simulink model "sampleModel7424_pp_1_1"  (R2018a)
settings: Solver=VariableStepAuto  StartTime=0.0  StopTime=10.0  RelTol=1e-3
undefined symbols (not defined in the file): DiscIntNeverNeededParam
libraries: simulink x211
(part 3 of 7)

== system sampleModel7424_pp_1_1/cfblk137 ==
  cfblk1 : Inport
  Action Port : ActionPort  ActionType=then
  cfblk10 : simulink/Discrete/Transfer Fcn Lead or Lag  PoleZ=0.95  ZeroZ=0.75  ICPrevOutput=0.0  ICPrevInput=0.0  DoSatur=off
      settings: SourceProductName=Simulink  SourceProductBaseCode=SL
  cfblk15 : Delay
  cfblk16 : Delay
  cfblk17 : DataTypeConversion  OutDataTypeStr=double
  cfblk18 : DataTypeConversion  OutDataTypeStr=double
  cfblk3 : Delay
  cfblk4 : DiscreteTransferFcn
  cfblk5 : DiscreteFilter
  cfblk6 : simulink/Discrete/Transfer Fcn Lead or Lag  PoleZ=0.95  ZeroZ=0.75  ICPrevOutput=0.0  ICPrevInput=0.0  DoSatur=off
      settings: SourceProductName=Simulink  SourceProductBaseCode=SL
  cfblk7 : Delay  DelayLengthSource=Input port
      settings: InputPortMap=u0,p1
  cfblk8 : simulink/Discrete/Tapped Delay  vinit=0.0  samptime=-1  NumDelays=1  DelayOrder=Oldest  includeCurrent=off
  cfblk9 : Delay  DelayLengthSource=Input port
      settings: InputPortMap=u0,p1
  cyemi_{473,475..476,479..482,485} (8 alike) : DataTypeConversion  OutDataTypeStr=double
  cyemi_{474,477..478,483..484,486} (6 alike) : DataTypeConversion  OutDataTypeStr=uint32
  cfblk2 : Outport
  cfblk11 : Outport  Port=2
  cfblk12 : Outport  Port=3
  cfblk13 : Outport  Port=4
  cfblk14 : Outport  Port=5
  wires:
  cfblk9/1 -> cfblk11/1, cyemi_482/1
  cfblk7/1 -> cfblk12/1
  cfblk6/1 -> cyemi_473/1, cyemi_485/1
  cfblk1/1 -> cfblk13/1
  cfblk3/1 -> cfblk14/1, cyemi_484/1
  cfblk8/1 -> cyemi_474/1, cyemi_477/1, cyemi_483/1, cyemi_486/1
  cfblk17/1 -> cfblk2/1
  cyemi_473/1 -> cfblk10/1
  cyemi_474/1 -> cfblk15/1
  cyemi_475/1 -> cfblk16/1
  cfblk10/1 -> cyemi_475/1
  cyemi_476/1 -> cfblk17/1
  cfblk4/1 -> cyemi_476/1
  cyemi_477/1 -> cfblk18/1
  cyemi_478/1 -> cfblk3/1
  cfblk15/1 -> cyemi_478/1
  cyemi_479/1 -> cfblk4/1
  cfblk18/1 -> cyemi_479/1
  cyemi_480/1 -> cfblk5/1
  cfblk16/1 -> cyemi_480/1
  cyemi_481/1 -> cfblk6/1
  cfblk5/1 -> cyemi_481/1
  cyemi_482/1 -> cfblk7/1
  cyemi_483/1 -> cfblk7/2
  cyemi_484/1 -> cfblk8/1
  cyemi_485/1 -> cfblk9/1
  cyemi_486/1 -> cfblk9/2

== system sampleModel7424_pp_1_1/cfblk138 ==
  cfblk1 : Inport
  cfblk6 : Inport  Port=2
  Action Port : ActionPort  ActionType=else
  cfblk3 : DiscreteTransferFcn
  cfblk4 : simulink/Continuous/PID Controller (2DOF)  Controller=PID  TimeDomain=Discrete-time  SampleTime=-1  IntegratorMethod=Forward Euler  FilterMethod=Forward Euler  Form=Parallel  UseFilter=on  ControllerParametersSource=internal  P=1  I=1  D=0  N=100  b=1  c=1  InitialConditionSource=internal  InitialConditionForIntegrator=0  InitialConditionForFilter=0  ExternalReset=none  LimitOutput=off  UpperSaturationLimit=inf  LowerSaturationLimit=-inf  LinearizeAsGain=off  AntiWindupMode=none  Kb=1  TrackingMode=off  Kt=1  PParamMin=[]  PParamMax=[]  IParamMin=[]  IParamMax=[]  DParamMin=[]  DParamMax=[]  NParamMin=[]  NParamMax=[]  bParamMin=[]  bParamMax=[]  cParamMin=[]  cParamMax=[]  KbParamMin=[]  KbParamMax=[]  KtParamMin=[]  KtParamMax=[]  POutMin=[]  POutMax=[]  IOutMin=[]  IOutMax=[]  DOutMin=[]  DOutMax=[]  NOutMin=[]  NOutMax=[]  bOutMin=[]  bOutMax=[]  cOutMin=[]  cOutMax=[]  KbOutMin=[]  KbOutMax=[]  KtOutMin=[]  KtOutMax=[]  IntegratorOutMin=[]  IntegratorOutMax=[]  FilterOutMin=[]  FilterOutMax=[]  SumOutMin=[]  SumOutMax=[]  Sum1OutMin=[]  Sum1OutMax=[]  Sum2OutMin=[]  Sum2OutMax=[]  Sum3OutMin=[]  Sum3OutMax=[]  SumI1OutMin=[]  SumI1OutMax=[]  SumI2OutMin=[]  SumI2OutMax=[]  SumI3OutMin=[]  SumI3OutMax=[]  SumDOutMin=[]  SumDOutMax=[]  SaturationOutMin=[]  SaturationOutMax=[]  IntegratorContinuousStateAttributes=''  IntegratorStateMustResolveToSignalObject=off  IntegratorRTWStateStorageClass=Auto  FilterContinuousStateAttributes=''  FilterStateMustResolveToSignalObject=off  FilterRTWStateStorageClass=Auto  DifferentiatorICPrevScaledInput=0  DifferentiatorOutMin=[]  DifferentiatorOutMax=[]  FilterDiffOutCoefMin=[]  FilterDiffOutCoefMax=[]  SumDenOutMin=[]  SumDenOutMax=[]  SumNumOutMin=[]  SumNumOutMax=[]  ReciprocalOutMin=[]  ReciprocalOutMax=[]  DivideOutMin=[]  DivideOutMax=[]  TunerSelectOption=Transfer Function Based (PID Tuner App)
  cfblk5 : DiscreteFilter
  cyemi_{489..492} (4 alike) : DataTypeConversion  OutDataTypeStr=double
  emi_{144,174,244,296} (4 alike) : UnaryMinus
  emi_145 : MATLAB Function  TreatAsAtomicUnit=on
  emi_175 : MATLAB Function  TreatAsAtomicUnit=on
  emi_245 : MATLAB Function  TreatAsAtomicUnit=on
  emi_297 : MATLAB Function  TreatAsAtomicUnit=on
  cfblk2 : Outport
  cfblk7 : Outport  Port=2
  wires:
  cfblk1/1 -> cfblk2/1
  cfblk5/1 -> cfblk7/1
  cyemi_489/1 -> cfblk3/1, emi_144/1, emi_145/1(o), emi_174/1, emi_175/1(o)
  cfblk4/1 -> cyemi_489/1
  cyemi_490/1 -> cfblk4/1, emi_296/1, emi_297/1(o)
  cfblk6/1 -> cyemi_490/1, cyemi_491/1
  cyemi_491/1 -> cfblk4/2
  cyemi_492/1 -> cfblk5/1, emi_244/1, emi_245/1(o)
  cfblk3/1 -> cyemi_492/1
  emi_144/1 -> emi_145/2(e)
  emi_174/1 -> emi_175/2(e)
  emi_244/1 -> emi_245/2(e)
  emi_296/1 -> emi_297/2(e)

== system sampleModel7424_pp_1_1/cfblk139 ==
  cfblk1 : Inport
  cfblk8 : Inport  Port=2
  Action Port : ActionPort  ActionType=then
  cfblk3 : DiscreteZeroPole  Poles=[0 0.5]  Gain=1  SampleTime=-1
  cfblk4 : DiscreteTransferFcn
  cfblk5 : DiscreteIntegrator  SampleTime=-1  OutDataTypeStr=double  ICPrevOutput=DiscIntNeverNeededParam  ICPrevScaledInput=DiscIntNeverNeededParam
  cfblk6 : simulink/Discrete/Tapped Delay  vinit=0.0  samptime=-1  NumDelays=1  DelayOrder=Oldest  includeCurrent=off
  cfblk7 : simulink/Discrete/Difference  ICPrevInput=0.0  OutMin=[]  OutMax=[]  OutDataTypeStr=double  OutputDataTypeScalingMode=double  OutDataType=fixdt(1, 16)  OutScaling=2^-10  DoSatur=off
  cyemi_{495..499} (5 alike) : DataTypeConversion  OutDataTypeStr=double
  cfblk2 : Outport
  cfblk9 : Outport  Port=2
  cfblk10 : Outport  Port=3
  wires:
  cfblk4/1 -> cyemi_495/1, cyemi_499/1
  cfblk3/1 -> cfblk9/1
  cfblk8/1 -> cfblk2/1
  cfblk7/1 -> cfblk10/1
  cyemi_495/1 -> cfblk3/1
  cyemi_496/1 -> cfblk4/1
  cfblk5/1 -> cyemi_496/1
  cyemi_497/1 -> cfblk5/1
  cfblk6/1 -> cyemi_497/1
  cyemi_498/1 -> cfblk6/1
  cfblk1/1 -> cyemi_498/1
  cyemi_499/1 -> cfblk7/1

== system sampleModel7424_pp_1_1/cfblk140 ==
  cfblk1 : Inport
  Action Port : ActionPort  ActionType=else
  cfblk3 : Delay
  cfblk4 : simulink/Discrete/Transfer Fcn First Order  PoleZ=0.95  ICPrevOutput=0.0  DoSatur=off
      settings: SourceProductName=Simulink
  cfblk5 : Delay  ShowEnablePort=on
      settings: InputPortMap=u0,e6
  cfblk6 : Delay  ShowEnablePort=on
      settings: InputPortMap=u0,e6
  cyemi_{502..507} (6 alike) : DataTypeConversion  OutDataTypeStr=double
  emi_118 : UnaryMinus
  emi_119 : MATLAB Function  TreatAsAtomicUnit=on
  emi_270 : UnaryMinus
  emi_271 : MATLAB Function  TreatAsAtomicUnit=on
  emi_304 : UnaryMinus
  emi_305 : MATLAB Function  TreatAsAtomicUnit=on
  cfblk2 : Outport
  cfblk7 : Outport  Port=2
  cfblk8 : Outport  Port=3
  wires:
  cfblk4/1 -> cyemi_505/1, cyemi_506/1
  cfblk3/1 -> cyemi_504/1, cyemi_507/1
  cfblk6/1 -> cfblk2/1
  cfblk1/1 -> cyemi_502/1, cyemi_503/1
  cfblk5/1 -> cfblk8/1, cfblk7/1
  cyemi_502/1 -> cfblk3/1, emi_118/1, emi_119/1(o), emi_270/1, emi_271/1(o)
  cyemi_503/1 -> cfblk4/1, emi_304/1, emi_305/1(o)
  cyemi_504/1 -> cfblk5/1
  cyemi_505/1 -> cfblk5/2
  cyemi_506/1 -> cfblk6/1
  cyemi_507/1 -> cfblk6/2
  emi_118/1 -> emi_119/2(e)
  emi_270/1 -> emi_271/2(e)
  emi_304/1 -> emi_305/2(e)

== system sampleModel7424_pp_1_1/cfblk141 ==
  cfblk1 : Inport
  cfblk13 : Inport  Port=2
  cfblk14 : Inport  Port=3
  Action Port : ActionPort  ActionType=then
  cfblk10 : DiscreteFilter
  cfblk11 : simulink/Discrete/Transfer Fcn Lead or Lag  PoleZ=0.95  ZeroZ=0.75  ICPrevOutput=0.0  ICPrevInput=0.0  DoSatur=off
      settings: SourceProductName=Simulink  SourceProductBaseCode=SL
  cfblk12 : simulink/Discrete/Transfer Fcn First Order  PoleZ=0.95  ICPrevOutput=0.0  DoSatur=off
      settings: SourceProductName=Simulink
  cfblk3 : DiscreteIntegrator  SampleTime=-1  OutDataTypeStr=double  ICPrevOutput=DiscIntNeverNeededParam  ICPrevScaledInput=DiscIntNeverNeededParam
  cfblk4 : simulink/Discrete/Transfer Fcn Lead or Lag  PoleZ=0.95  ZeroZ=0.75  ICPrevOutput=0.0  ICPrevInput=0.0  DoSatur=off
      settings: SourceProductName=Simulink  SourceProductBaseCode=SL
  cfblk5 : DiscreteIntegrator  SampleTime=-1  OutDataTypeStr=double  ICPrevOutput=DiscIntNeverNeededParam  ICPrevScaledInput=DiscIntNeverNeededParam
  cfblk6 : simulink/Discrete/Transfer Fcn First Order  PoleZ=0.95  ICPrevOutput=0.0  DoSatur=off
      settings: SourceProductName=Simulink
  cfblk7 : simulink/Continuous/PID Controller  Controller=PID  TimeDomain=Discrete-time  SampleTime=-1  IntegratorMethod=Forward Euler  FilterMethod=Forward Euler  Form=Parallel  UseFilter=on  ControllerParametersSource=internal  P=1  I=1  D=0  N=100  InitialConditionSource=internal  InitialConditionForIntegrator=0  InitialConditionForFilter=0  ExternalReset=none  LimitOutput=off  UpperSaturationLimit=inf  LowerSaturationLimit=-inf  LinearizeAsGain=off  AntiWindupMode=none  Kb=1  TrackingMode=off  Kt=1  PParamMin=[]  PParamMax=[]  IParamMin=[]  IParamMax=[]  DParamMin=[]  DParamMax=[]  NParamMin=[]  NParamMax=[]  KbParamMin=[]  KbParamMax=[]  KtParamMin=[]  KtParamMax=[]  POutMin=[]  POutMax=[]  IOutMin=[]  IOutMax=[]  DOutMin=[]  DOutMax=[]  NOutMin=[]  NOutMax=[]  KbOutMin=[]  KbOutMax=[]  KtOutMin=[]  KtOutMax=[]  IntegratorOutMin=[]  IntegratorOutMax=[]  FilterOutMin=[]  FilterOutMax=[]  SumOutMin=[]  SumOutMax=[]  SumI1OutMin=[]  SumI1OutMax=[]  SumI2OutMin=[]  SumI2OutMax=[]  SumI3OutMin=[]  SumI3OutMax=[]  SumDOutMin=[]  SumDOutMax=[]  SaturationOutMin=[]  SaturationOutMax=[]  IntegratorContinuousStateAttributes=''  IntegratorStateMustResolveToSignalObject=off  IntegratorRTWStateStorageClass=Auto  FilterContinuousStateAttributes=''  FilterStateMustResolveToSignalObject=off  FilterRTWStateStorageClass=Auto  DifferentiatorICPrevScaledInput=0  DifferentiatorOutMin=[]  DifferentiatorOutMax=[]  FilterDiffOutCoefMin=[]  FilterDiffOutCoefMax=[]  SumDenOutMin=[]  SumDenOutMax=[]  SumNumOutMin=[]  SumNumOutMax=[]  ReciprocalOutMin=[]  ReciprocalOutMax=[]  DivideOutMin=[]  DivideOutMax=[]  TunerSelectOption=Transfer Function Based (PID Tuner App)
  cfblk8 : simulink/Discrete/Transfer Fcn Real Zero  ZeroZ=0.75  ICPrevInput=0.0  DoSatur=off
      settings: SourceProductName=Simulink  SourceProductBaseCode=SL
  cfblk9 : DiscreteZeroPole  Poles=[0 0.5]  Gain=1  SampleTime=-1
  cyemi_{511..520} (10 alike) : DataTypeConversion  OutDataTypeStr=double
  emi_{142,216,242,262} (4 alike) : UnaryMinus
  emi_143 : MATLAB Function  TreatAsAtomicUnit=on
  emi_217 : MATLAB Function  TreatAsAtomicUnit=on
  emi_243 : MATLAB Function  TreatAsAtomicUnit=on
  emi_263 : MATLAB Function  TreatAsAtomicUnit=on
  cfblk2 : Outport
  wires:
  cfblk12/1 -> cfblk2/1
  cyemi_511/1 -> cfblk10/1, emi_142/1, emi_143/1(o)
  cfblk4/1 -> cyemi_511/1
  cyemi_512/1 -> cfblk11/1
  cfblk7/1 -> cyemi_512/1
  cyemi_513/1 -> cfblk12/1
  cfblk13/1 -> cyemi_513/1
  cyemi_514/1 -> cfblk3/1
  cfblk9/1 -> cyemi_514/1
  cyemi_515/1 -> cfblk4/1
  cfblk6/1 -> cyemi_515/1
  cyemi_516/1 -> cfblk5/1, emi_242/1, emi_243/1(o)
  cfblk11/1 -> cyemi_516/1
  cyemi_517/1 -> cfblk6/1, emi_216/1, emi_217/1(o)
  cfblk14/1 -> cyemi_517/1
  cyemi_518/1 -> cfblk7/1
  cfblk10/1 -> cyemi_518/1
  cyemi_519/1 -> cfblk8/1, emi_262/1, emi_263/1(o)
  cfblk3/1 -> cyemi_519/1
  cyemi_520/1 -> cfblk9/1
  cfblk1/1 -> cyemi_520/1
  emi_142/1 -> emi_143/2(e)
  emi_216/1 -> emi_217/2(e)
  emi_242/1 -> emi_243/2(e)
  emi_262/1 -> emi_263/2(e)

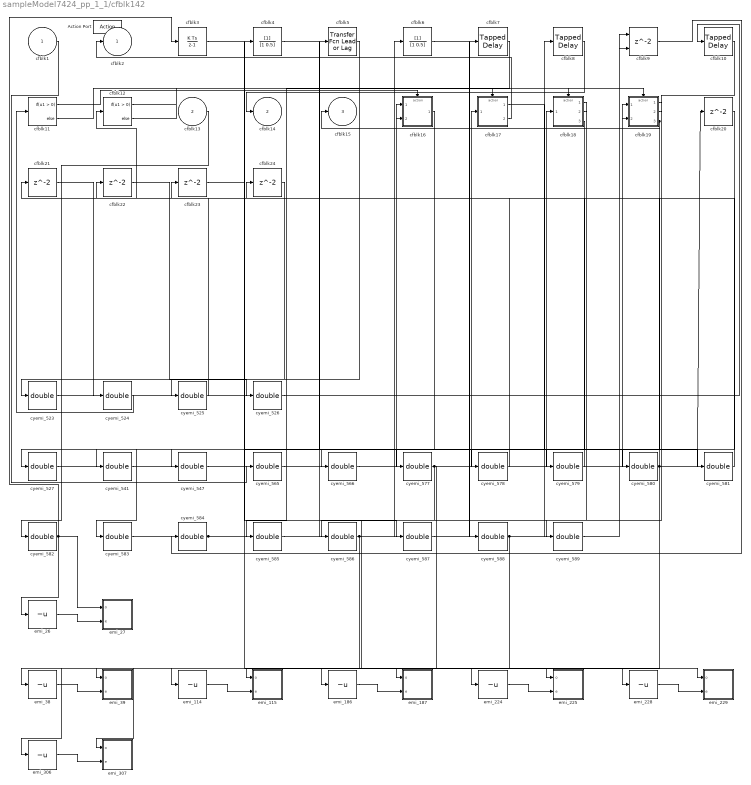
== system sampleModel7424_pp_1_1/cfblk142 ==
  cfblk1 : Inport
  cfblk13 : Inport  Port=2
  Action Port : ActionPort  ActionType=else
  cfblk10 : simulink/Discrete/Tapped Delay  vinit=0.0  samptime=-1  NumDelays=1  DelayOrder=Oldest  includeCurrent=off
  cfblk11 : If  SampleTime=1
  cfblk12 : If  SampleTime=1
  cfblk16 : Subsystem  TreatAsAtomicUnit=on
  cfblk17 : Subsystem  TreatAsAtomicUnit=on
  cfblk18 : Subsystem  TreatAsAtomicUnit=on
  cfblk19 : Subsystem  TreatAsAtomicUnit=on
  cfblk{20..24} (5 alike) : Delay
  cfblk3 : DiscreteIntegrator  SampleTime=-1  OutDataTypeStr=double  ICPrevOutput=DiscIntNeverNeededParam  ICPrevScaledInput=DiscIntNeverNeededParam
  cfblk4 : DiscreteFilter
  cfblk5 : simulink/Discrete/Transfer Fcn Lead or Lag  PoleZ=0.95  ZeroZ=0.75  ICPrevOutput=0.0  ICPrevInput=0.0  DoSatur=off
      settings: SourceProductName=Simulink  SourceProductBaseCode=SL
  cfblk6 : DiscreteFilter
  cfblk7 : simulink/Discrete/Tapped Delay  vinit=0.0  samptime=-1  NumDelays=1  DelayOrder=Oldest  includeCurrent=off
  cfblk8 : simulink/Discrete/Tapped Delay  vinit=0.0  samptime=-1  NumDelays=1  DelayOrder=Oldest  includeCurrent=off
  cfblk9 : Delay  ShowEnablePort=on
      settings: InputPortMap=u0,e6
  cyemi_{523..527,541,547,565..566,577..589} (22 alike) : DataTypeConversion  OutDataTypeStr=double
  emi_{26,38,114,186,224,228,306} (7 alike) : UnaryMinus
  emi_115 : MATLAB Function  TreatAsAtomicUnit=on
  emi_187 : MATLAB Function  TreatAsAtomicUnit=on
  emi_225 : MATLAB Function  TreatAsAtomicUnit=on
  emi_229 : MATLAB Function  TreatAsAtomicUnit=on
  emi_27 : MATLAB Function  TreatAsAtomicUnit=on
  emi_307 : MATLAB Function  TreatAsAtomicUnit=on
  emi_39 : MATLAB Function  TreatAsAtomicUnit=on
  cfblk2 : Outport
  cfblk14 : Outport  Port=2
  cfblk15 : Outport  Port=3
  wires:
  cfblk8/1 -> cfblk14/1
  cfblk19/3(cfblk13) -> cfblk15/1, cyemi_582/1
  cfblk17/2(cfblk7) -> cfblk2/1
  cfblk11/1 -> cfblk16/Action
  cfblk11/2 -> cfblk17/Action
  cfblk12/1 -> cfblk18/Action
  cfblk12/2 -> cfblk19/Action
  cyemi_523/1 -> cfblk10/1
  cfblk5/1 -> cyemi_523/1
  cyemi_524/1 -> cfblk11/1
  cfblk21/1 -> cyemi_524/1
  cyemi_525/1 -> cfblk12/1
  cfblk24/1 -> cyemi_525/1
  cyemi_526/1 -> cfblk16/1(cfblk1)
  cfblk22/1 -> cyemi_526/1
  cyemi_527/1 -> cfblk16/2(cfblk11)
  cfblk13/1 -> cyemi_527/1
  cyemi_541/1 -> cfblk17/1(cfblk1)
  cfblk19/1(cfblk2) -> cyemi_541/1
  cyemi_547/1 -> cfblk18/1(cfblk1)
  cfblk20/1 -> cyemi_547/1
  cyemi_565/1 -> cfblk19/1(cfblk1)
  cfblk1/1 -> cyemi_565/1
  cyemi_566/1 -> cfblk19/2(cfblk11)
  cfblk23/1 -> cyemi_566/1
  cyemi_577/1 -> cfblk20/1, emi_186/1, emi_187/1(o)
  cfblk16/1(cfblk2) -> cyemi_577/1
  cyemi_578/1 -> cfblk21/1
  cfblk10/1 -> cyemi_578/1
  cyemi_579/1 -> cfblk22/1
  cfblk18/2(cfblk14) -> cyemi_579/1
  cyemi_580/1 -> cfblk23/1, emi_224/1, emi_225/1(o), emi_306/1, emi_307/1(o)
  cfblk4/1 -> cyemi_580/1
  cyemi_581/1 -> cfblk24/1
  cfblk17/1(cfblk2) -> cyemi_581/1
  cyemi_582/1 -> cfblk3/1, emi_26/1, emi_27/1(o)
  cyemi_583/1 -> cfblk4/1
  cfblk18/3(cfblk15) -> cyemi_583/1
  cyemi_584/1 -> cfblk5/1, emi_228/1, emi_229/1(o)
  cfblk9/1 -> cyemi_584/1
  cyemi_585/1 -> cfblk6/1
  cfblk7/1 -> cyemi_585/1
  cyemi_586/1 -> cfblk7/1, emi_114/1, emi_115/1(o)
  cfblk19/2(cfblk12) -> cyemi_586/1
  cyemi_587/1 -> cfblk8/1
  cfblk3/1 -> cyemi_587/1
  cyemi_588/1 -> cfblk9/1, emi_38/1, emi_39/1(o)
  cfblk6/1 -> cyemi_588/1
  cyemi_589/1 -> cfblk9/2
  cfblk18/1(cfblk2) -> cyemi_589/1
  emi_26/1 -> emi_27/2(e)
  emi_38/1 -> emi_39/2(e)
  emi_114/1 -> emi_115/2(e)
  emi_186/1 -> emi_187/2(e)
  emi_224/1 -> emi_225/2(e)
  emi_228/1 -> emi_229/2(e)
  emi_306/1 -> emi_307/2(e)

== system sampleModel7424_pp_1_1/cfblk143 ==
  cfblk1 : Inport
  Action Port : ActionPort  ActionType=then
  cfblk3 : UnitDelay  SampleTime=-1
  cfblk4 : DiscreteZeroPole  Poles=[0 0.5]  Gain=1  SampleTime=-1
  cfblk5 : DiscreteZeroPole  Poles=[0 0.5]  Gain=1  SampleTime=-1
  cfblk6 : simulink/Discrete/Transfer Fcn First Order  PoleZ=0.95  ICPrevOutput=0.0  DoSatur=off
      settings: SourceProductName=Simulink
  cfblk7 : DiscreteZeroPole  Poles=[0 0.5]  Gain=1  SampleTime=-1
  cfblk8 : Delay
  cfblk9 : DataTypeConversion  OutDataTypeStr=double
  cyemi_{591..596} (6 alike) : DataTypeConversion  OutDataTypeStr=double
  cyemi_597 : DataTypeConversion  OutDataTypeStr=uint16
  cfblk2 : Outport
  wires:
  cfblk7/1 -> cfblk2/1
  cyemi_591/1 -> cfblk3/1
  cfblk8/1 -> cyemi_591/1
  cyemi_592/1 -> cfblk4/1
  cfblk6/1 -> cyemi_592/1
  cyemi_593/1 -> cfblk5/1
  cfblk4/1 -> cyemi_593/1
  cyemi_594/1 -> cfblk6/1
  cfblk3/1 -> cyemi_594/1
  cyemi_595/1 -> cfblk7/1
  cfblk9/1 -> cyemi_595/1
  cyemi_596/1 -> cfblk8/1
  cfblk5/1 -> cyemi_596/1
  cyemi_597/1 -> cfblk9/1
  cfblk1/1 -> cyemi_597/1

== system sampleModel7424_pp_1_1/cfblk144 ==
  cfblk1 : Inport
  cfblk12 : Inport  Port=2
  cfblk13 : Inport  Port=3
  Action Port : ActionPort  ActionType=else
  cfblk10 : simulink/Continuous/PID Controller  Controller=PID  TimeDomain=Discrete-time  SampleTime=-1  IntegratorMethod=Forward Euler  FilterMethod=Forward Euler  Form=Parallel  UseFilter=on  ControllerParametersSource=internal  P=1  I=1  D=0  N=100  InitialConditionSource=internal  InitialConditionForIntegrator=0  InitialConditionForFilter=0  ExternalReset=none  LimitOutput=off  UpperSaturationLimit=inf  LowerSaturationLimit=-inf  LinearizeAsGain=off  AntiWindupMode=none  Kb=1  TrackingMode=off  Kt=1  PParamMin=[]  PParamMax=[]  IParamMin=[]  IParamMax=[]  DParamMin=[]  DParamMax=[]  NParamMin=[]  NParamMax=[]  KbParamMin=[]  KbParamMax=[]  KtParamMin=[]  KtParamMax=[]  POutMin=[]  POutMax=[]  IOutMin=[]  IOutMax=[]  DOutMin=[]  DOutMax=[]  NOutMin=[]  NOutMax=[]  KbOutMin=[]  KbOutMax=[]  KtOutMin=[]  KtOutMax=[]  IntegratorOutMin=[]  IntegratorOutMax=[]  FilterOutMin=[]  FilterOutMax=[]  SumOutMin=[]  SumOutMax=[]  SumI1OutMin=[]  SumI1OutMax=[]  SumI2OutMin=[]  SumI2OutMax=[]  SumI3OutMin=[]  SumI3OutMax=[]  SumDOutMin=[]  SumDOutMax=[]  SaturationOutMin=[]  SaturationOutMax=[]  IntegratorContinuousStateAttributes=''  IntegratorStateMustResolveToSignalObject=off  IntegratorRTWStateStorageClass=Auto  FilterContinuousStateAttributes=''  FilterStateMustResolveToSignalObject=off  FilterRTWStateStorageClass=Auto  DifferentiatorICPrevScaledInput=0  DifferentiatorOutMin=[]  DifferentiatorOutMax=[]  FilterDiffOutCoefMin=[]  FilterDiffOutCoefMax=[]  SumDenOutMin=[]  SumDenOutMax=[]  SumNumOutMin=[]  SumNumOutMax=[]  ReciprocalOutMin=[]  ReciprocalOutMax=[]  DivideOutMin=[]  DivideOutMax=[]  TunerSelectOption=Transfer Function Based (PID Tuner App)
  cfblk11 : Delay  DelayLengthSource=Input port
      settings: InputPortMap=u0,p1
  cfblk14 : Delay
  cfblk3 : simulink/Discrete/Tapped Delay  vinit=0.0  samptime=-1  NumDelays=1  DelayOrder=Oldest  includeCurrent=off
  cfblk4 : simulink/Continuous/PID Controller  Controller=PID  TimeDomain=Discrete-time  SampleTime=-1  IntegratorMethod=Forward Euler  FilterMethod=Forward Euler  Form=Parallel  UseFilter=on  ControllerParametersSource=internal  P=1  I=1  D=0  N=100  InitialConditionSource=internal  InitialConditionForIntegrator=0  InitialConditionForFilter=0  ExternalReset=none  LimitOutput=off  UpperSaturationLimit=inf  LowerSaturationLimit=-inf  LinearizeAsGain=off  AntiWindupMode=none  Kb=1  TrackingMode=off  Kt=1  PParamMin=[]  PParamMax=[]  IParamMin=[]  IParamMax=[]  DParamMin=[]  DParamMax=[]  NParamMin=[]  NParamMax=[]  KbParamMin=[]  KbParamMax=[]  KtParamMin=[]  KtParamMax=[]  POutMin=[]  POutMax=[]  IOutMin=[]  IOutMax=[]  DOutMin=[]  DOutMax=[]  NOutMin=[]  NOutMax=[]  KbOutMin=[]  KbOutMax=[]  KtOutMin=[]  KtOutMax=[]  IntegratorOutMin=[]  IntegratorOutMax=[]  FilterOutMin=[]  FilterOutMax=[]  SumOutMin=[]  SumOutMax=[]  SumI1OutMin=[]  SumI1OutMax=[]  SumI2OutMin=[]  SumI2OutMax=[]  SumI3OutMin=[]  SumI3OutMax=[]  SumDOutMin=[]  SumDOutMax=[]  SaturationOutMin=[]  SaturationOutMax=[]  IntegratorContinuousStateAttributes=''  IntegratorStateMustResolveToSignalObject=off  IntegratorRTWStateStorageClass=Auto  FilterContinuousStateAttributes=''  FilterStateMustResolveToSignalObject=off  FilterRTWStateStorageClass=Auto  DifferentiatorICPrevScaledInput=0  DifferentiatorOutMin=[]  DifferentiatorOutMax=[]  FilterDiffOutCoefMin=[]  FilterDiffOutCoefMax=[]  SumDenOutMin=[]  SumDenOutMax=[]  SumNumOutMin=[]  SumNumOutMax=[]  ReciprocalOutMin=[]  ReciprocalOutMax=[]  DivideOutMin=[]  DivideOutMax=[]  TunerSelectOption=Transfer Function Based (PID Tuner App)
  cfblk5 : simulink/Discrete/Transfer Fcn Real Zero  ZeroZ=0.75  ICPrevInput=0.0  DoSatur=off
      settings: SourceProductName=Simulink  SourceProductBaseCode=SL
  cfblk6 : DiscreteFir
  cfblk7 : DiscreteFir
  cfblk8 : DiscreteTransferFcn
  cfblk9 : simulink/Discrete/Transfer Fcn Lead or Lag  PoleZ=0.95  ZeroZ=0.75  ICPrevOutput=0.0  ICPrevInput=0.0  DoSatur=off
      settings: SourceProductName=Simulink  SourceProductBaseCode=SL
  cyemi_{601..611} (11 alike) : DataTypeConversion  OutDataTypeStr=double
  emi_196 : UnaryMinus
  emi_197 : MATLAB Function  TreatAsAtomicUnit=on
  cfblk2 : Outport
  wires:
  cfblk12/1 -> cfblk2/1
  cyemi_601/1 -> cfblk10/1
  cfblk5/1 -> cyemi_601/1
  cyemi_602/1 -> cfblk11/1
  cfblk1/1 -> cyemi_602/1
  cyemi_603/1 -> cfblk11/2
  cfblk3/1 -> cyemi_603/1
  cyemi_604/1 -> cfblk14/1
  cfblk7/1 -> cyemi_604/1
  cyemi_605/1 -> cfblk3/1
  cfblk9/1 -> cyemi_605/1
  cyemi_606/1 -> cfblk4/1, emi_196/1, emi_197/1(o)
  cfblk13/1 -> cyemi_606/1
  cyemi_607/1 -> cfblk5/1
  cfblk4/1 -> cyemi_607/1
  cyemi_608/1 -> cfblk6/1
  cfblk14/1 -> cyemi_608/1
  cyemi_609/1 -> cfblk7/1
  cfblk8/1 -> cyemi_609/1
  cyemi_610/1 -> cfblk8/1
  cfblk6/1 -> cyemi_610/1
  cyemi_611/1 -> cfblk9/1
  cfblk10/1 -> cyemi_611/1
  emi_196/1 -> emi_197/2(e)

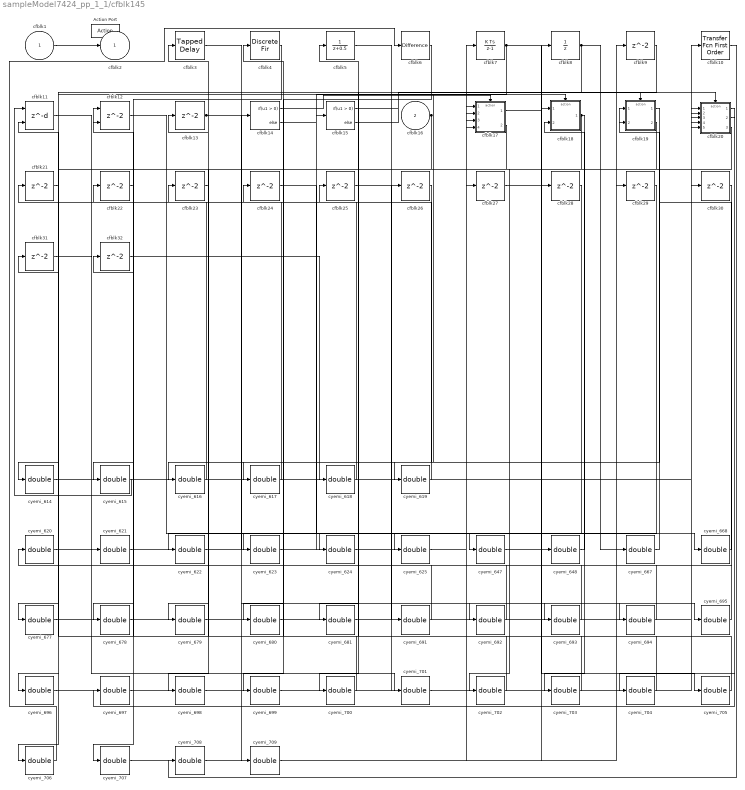
== system sampleModel7424_pp_1_1/cfblk145 ==
  cfblk1 : Inport
  cfblk16 : Inport  Port=2
  Action Port : ActionPort  ActionType=then
  cfblk10 : simulink/Discrete/Transfer Fcn First Order  PoleZ=0.95  ICPrevOutput=0.0  DoSatur=off
      settings: SourceProductName=Simulink
  cfblk11 : Delay  DelayLengthSource=Input port
      settings: InputPortMap=u0,p1
  cfblk12 : Delay  ShowEnablePort=on
      settings: InputPortMap=u0,e6
  cfblk{9,13,21..32} (14 alike) : Delay
  cfblk14 : If  SampleTime=1
  cfblk15 : If  SampleTime=1
  cfblk17 : Subsystem  TreatAsAtomicUnit=on
  cfblk18 : Subsystem  TreatAsAtomicUnit=on
  cfblk19 : Subsystem  TreatAsAtomicUnit=on
  cfblk20 : Subsystem  TreatAsAtomicUnit=on
  cfblk3 : simulink/Discrete/Tapped Delay  vinit=0.0  samptime=-1  NumDelays=1  DelayOrder=Oldest  includeCurrent=off
  cfblk4 : DiscreteFir
  cfblk5 : DiscreteTransferFcn
  cfblk6 : simulink/Discrete/Difference  ICPrevInput=0.0  OutMin=[]  OutMax=[]  OutDataTypeStr=double  OutputDataTypeScalingMode=double  OutDataType=fixdt(1, 16)  OutScaling=2^-10  DoSatur=off
  cfblk7 : DiscreteIntegrator  SampleTime=-1  OutDataTypeStr=double  ICPrevOutput=DiscIntNeverNeededParam  ICPrevScaledInput=DiscIntNeverNeededParam
  cfblk8 : UnitDelay  SampleTime=-1
  cyemi_{614..625,647..648,667..668,677..681,691..709} (40 alike) : DataTypeConversion  OutDataTypeStr=double
  cfblk2 : Outport
  wires:
  cfblk1/1 -> cfblk2/1
  cfblk8/1 -> cyemi_667/1, cyemi_681/1
  cfblk16/1 -> cyemi_615/1, cyemi_680/1
  cfblk13/1 -> cyemi_692/1, cyemi_693/1, cyemi_694/1
  cfblk7/1 -> cyemi_619/1, cyemi_695/1, cyemi_696/1
  cfblk18/1(cfblk2) -> cyemi_614/1, cyemi_624/1, cyemi_703/1
  cfblk14/1 -> cfblk17/Action
  cfblk14/2 -> cfblk18/Action
  cfblk15/1 -> cfblk19/Action
  cfblk15/2 -> cfblk20/Action
  cyemi_614/1 -> cfblk10/1
  cyemi_615/1 -> cfblk11/1
  cyemi_616/1 -> cfblk11/2
  cfblk19/1(cfblk2) -> cyemi_616/1
  cyemi_617/1 -> cfblk12/1
  cfblk6/1 -> cyemi_617/1
  cyemi_618/1 -> cfblk12/2
  cfblk32/1 -> cyemi_618/1
  cyemi_619/1 -> cfblk13/1
  cyemi_620/1 -> cfblk14/1
  cfblk30/1 -> cyemi_620/1
  cyemi_621/1 -> cfblk15/1
  cfblk31/1 -> cyemi_621/1
  cyemi_622/1 -> cfblk17/1(cfblk1)
  cfblk28/1 -> cyemi_622/1
  cyemi_623/1 -> cfblk17/2(cfblk14)
  cfblk26/1 -> cyemi_623/1
  cyemi_624/1 -> cfblk17/3(cfblk15)
  cyemi_625/1 -> cfblk17/4(cfblk16)
  cfblk24/1 -> cyemi_625/1
  cyemi_647/1 -> cfblk18/1(cfblk1)
  cfblk12/1 -> cyemi_647/1
  cyemi_648/1 -> cfblk18/2(cfblk15)
  cfblk27/1 -> cyemi_648/1
  cyemi_667/1 -> cfblk19/1(cfblk1)
  cyemi_668/1 -> cfblk19/2(cfblk11)
  cfblk25/1 -> cyemi_668/1
  cyemi_677/1 -> cfblk20/1(cfblk1)
  cfblk21/1 -> cyemi_677/1
  cyemi_678/1 -> cfblk20/2(cfblk10)
  cfblk22/1 -> cyemi_678/1
  cyemi_679/1 -> cfblk20/3(cfblk11)
  cfblk23/1 -> cyemi_679/1
  cyemi_680/1 -> cfblk20/4(cfblk12)
  cyemi_681/1 -> cfblk20/5(cfblk13)
  cyemi_691/1 -> cfblk21/1
  cfblk5/1 -> cyemi_691/1
  cyemi_692/1 -> cfblk22/1
  cyemi_693/1 -> cfblk23/1
  cyemi_694/1 -> cfblk24/1
  cyemi_695/1 -> cfblk25/1
  cyemi_696/1 -> cfblk26/1
  cyemi_697/1 -> cfblk27/1
  cfblk20/2(cfblk14) -> cyemi_697/1
  cyemi_698/1 -> cfblk28/1
  cfblk20/3(cfblk15) -> cyemi_698/1
  cyemi_699/1 -> cfblk29/1
  cfblk17/2(cfblk17) -> cyemi_699/1
  cyemi_700/1 -> cfblk3/1
  cfblk29/1 -> cyemi_700/1
  cyemi_701/1 -> cfblk30/1
  cfblk11/1 -> cyemi_701/1
  cyemi_702/1 -> cfblk31/1
  cfblk19/2(cfblk12) -> cyemi_702/1
  cyemi_703/1 -> cfblk32/1
  cyemi_704/1 -> cfblk4/1
  cfblk20/1(cfblk2) -> cyemi_704/1
  cyemi_705/1 -> cfblk5/1
  cfblk17/1(cfblk2) -> cyemi_705/1
  cyemi_706/1 -> cfblk6/1
  cfblk9/1 -> cyemi_706/1
  cyemi_707/1 -> cfblk7/1
  cfblk4/1 -> cyemi_707/1
  cyemi_708/1 -> cfblk8/1
  cfblk10/1 -> cyemi_708/1
  cyemi_709/1 -> cfblk9/1
  cfblk3/1 -> cyemi_709/1

== system sampleModel7424_pp_1_1/cfblk146 ==
  cfblk1 : Inport
  cfblk10 : Inport  Port=2
  Action Port : ActionPort  ActionType=else
  cfblk3 : UnitDelay  SampleTime=-1
  cfblk4 : DiscreteFilter
  cfblk5 : DiscreteZeroPole  Poles=[0 0.5]  Gain=1  SampleTime=-1
  cfblk6 : simulink/Discrete/Difference  ICPrevInput=0.0  OutMin=[]  OutMax=[]  OutDataTypeStr=double  OutputDataTypeScalingMode=double  OutDataType=fixdt(1, 16)  OutScaling=2^-10  DoSatur=off
  cfblk7 : simulink/Discrete/Difference  ICPrevInput=0.0  OutMin=[]  OutMax=[]  OutDataTypeStr=double  OutputDataTypeScalingMode=double  OutDataType=fixdt(1, 16)  OutScaling=2^-10  DoSatur=off
  cfblk8 : DiscreteFir
  cfblk9 : simulink/Continuous/PID Controller (2DOF)  Controller=PID  TimeDomain=Discrete-time  SampleTime=-1  IntegratorMethod=Forward Euler  FilterMethod=Forward Euler  Form=Parallel  UseFilter=on  ControllerParametersSource=internal  P=1  I=1  D=0  N=100  b=1  c=1  InitialConditionSource=internal  InitialConditionForIntegrator=0  InitialConditionForFilter=0  ExternalReset=none  LimitOutput=off  UpperSaturationLimit=inf  LowerSaturationLimit=-inf  LinearizeAsGain=off  AntiWindupMode=none  Kb=1  TrackingMode=off  Kt=1  PParamMin=[]  PParamMax=[]  IParamMin=[]  IParamMax=[]  DParamMin=[]  DParamMax=[]  NParamMin=[]  NParamMax=[]  bParamMin=[]  bParamMax=[]  cParamMin=[]  cParamMax=[]  KbParamMin=[]  KbParamMax=[]  KtParamMin=[]  KtParamMax=[]  POutMin=[]  POutMax=[]  IOutMin=[]  IOutMax=[]  DOutMin=[]  DOutMax=[]  NOutMin=[]  NOutMax=[]  bOutMin=[]  bOutMax=[]  cOutMin=[]  cOutMax=[]  KbOutMin=[]  KbOutMax=[]  KtOutMin=[]  KtOutMax=[]  IntegratorOutMin=[]  IntegratorOutMax=[]  FilterOutMin=[]  FilterOutMax=[]  SumOutMin=[]  SumOutMax=[]  Sum1OutMin=[]  Sum1OutMax=[]  Sum2OutMin=[]  Sum2OutMax=[]  Sum3OutMin=[]  Sum3OutMax=[]  SumI1OutMin=[]  SumI1OutMax=[]  SumI2OutMin=[]  SumI2OutMax=[]  SumI3OutMin=[]  SumI3OutMax=[]  SumDOutMin=[]  SumDOutMax=[]  SaturationOutMin=[]  SaturationOutMax=[]  IntegratorContinuousStateAttributes=''  IntegratorStateMustResolveToSignalObject=off  IntegratorRTWStateStorageClass=Auto  FilterContinuousStateAttributes=''  FilterStateMustResolveToSignalObject=off  FilterRTWStateStorageClass=Auto  DifferentiatorICPrevScaledInput=0  DifferentiatorOutMin=[]  DifferentiatorOutMax=[]  FilterDiffOutCoefMin=[]  FilterDiffOutCoefMax=[]  SumDenOutMin=[]  SumDenOutMax=[]  SumNumOutMin=[]  SumNumOutMax=[]  ReciprocalOutMin=[]  ReciprocalOutMax=[]  DivideOutMin=[]  DivideOutMax=[]  TunerSelectOption=Transfer Function Based (PID Tuner App)
  cyemi_{712..719} (8 alike) : DataTypeConversion  OutDataTypeStr=double
  cfblk2 : Outport
  cfblk11 : Outport  Port=2
  cfblk12 : Outport  Port=3
  wires:
  cfblk8/1 -> cfblk2/1
  cfblk4/1 -> cyemi_714/1, cyemi_719/1
  cfblk9/1 -> cfblk11/1
  cfblk6/1 -> cfblk12/1
  cfblk5/1 -> cyemi_712/1, cyemi_718/1
  cyemi_712/1 -> cfblk3/1
  cyemi_713/1 -> cfblk4/1
  cfblk10/1 -> cyemi_713/1
  cyemi_714/1 -> cfblk5/1
  cyemi_715/1 -> cfblk6/1
  cfblk7/1 -> cyemi_715/1
  cyemi_716/1 -> cfblk7/1
  cfblk3/1 -> cyemi_716/1
  cyemi_717/1 -> cfblk8/1
  cfblk1/1 -> cyemi_717/1
  cyemi_718/1 -> cfblk9/1
  cyemi_719/1 -> cfblk9/2

== system sampleModel7424_pp_1_1/cfblk147 ==
  cfblk1 : Inport
  cfblk10 : Inport  Port=2
  cfblk11 : Inport  Port=3
  Action Port : ActionPort  ActionType=then
  cfblk13 : Delay
  cfblk3 : DiscreteZeroPole  Poles=[0 0.5]  Gain=1  SampleTime=-1
  cfblk4 : Delay  DelayLengthSource=Input port
      settings: InputPortMap=u0,p1
  cfblk5 : DiscreteFilter
  cfblk6 : simulink/Discrete/Transfer Fcn First Order  PoleZ=0.95  ICPrevOutput=0.0  DoSatur=off
      settings: SourceProductName=Simulink
  cfblk7 : DiscreteFilter
  cfblk8 : DiscreteFilter
  cfblk9 : simulink/Discrete/Transfer Fcn Lead or Lag  PoleZ=0.95  ZeroZ=0.75  ICPrevOutput=0.0  ICPrevInput=0.0  DoSatur=off
      settings: SourceProductName=Simulink  SourceProductBaseCode=SL
  cyemi_{723..731} (9 alike) : DataTypeConversion  OutDataTypeStr=double
  emi_158 : UnaryMinus
  emi_159 : MATLAB Function  TreatAsAtomicUnit=on
  emi_36 : UnaryMinus
  emi_37 : MATLAB Function  TreatAsAtomicUnit=on
  emi_78 : UnaryMinus
  emi_79 : MATLAB Function  TreatAsAtomicUnit=on
  cfblk2 : Outport
  cfblk12 : Outport  Port=2
  wires:
  cfblk3/1 -> cfblk2/1
  cfblk7/1 -> cfblk12/1
  cyemi_723/1 -> cfblk13/1
  cfblk8/1 -> cyemi_723/1
  cyemi_724/1 -> cfblk3/1, emi_36/1, emi_37/1(o)
  cfblk5/1 -> cyemi_724/1
  cyemi_725/1 -> cfblk4/1
  cfblk13/1 -> cyemi_725/1
  cyemi_726/1 -> cfblk4/2
  cfblk9/1 -> cyemi_726/1
  cyemi_727/1 -> cfblk5/1, emi_78/1, emi_79/1(o)
  cfblk10/1 -> cyemi_727/1
  cyemi_728/1 -> cfblk6/1
  cfblk4/1 -> cyemi_728/1
  cyemi_729/1 -> cfblk7/1
  cfblk11/1 -> cyemi_729/1
  cyemi_730/1 -> cfblk8/1, emi_158/1, emi_159/1(o)
  cfblk6/1 -> cyemi_730/1
  cyemi_731/1 -> cfblk9/1
  cfblk1/1 -> cyemi_731/1
  emi_36/1 -> emi_37/2(e)
  emi_78/1 -> emi_79/2(e)
  emi_158/1 -> emi_159/2(e)

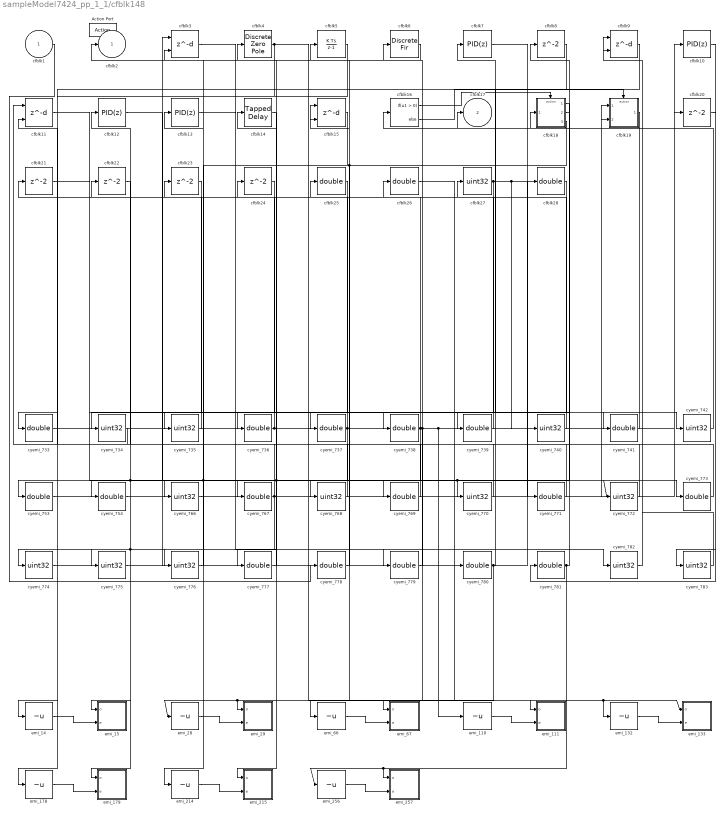
== system sampleModel7424_pp_1_1/cfblk148 ==
  cfblk1 : Inport
  Action Port : ActionPort  ActionType=else
  cfblk{7,10,12..13} (4 alike) : simulink/Continuous/PID Controller  Controller=PID  TimeDomain=Discrete-time  SampleTime=-1  IntegratorMethod=Forward Euler  FilterMethod=Forward Euler  Form=Parallel  UseFilter=on  ControllerParametersSource=internal  P=1  I=1  D=0  N=100  InitialConditionSource=internal  InitialConditionForIntegrator=0  InitialConditionForFilter=0  ExternalReset=none  LimitOutput=off  UpperSaturationLimit=inf  LowerSaturationLimit=-inf  LinearizeAsGain=off  AntiWindupMode=none  Kb=1  TrackingMode=off  Kt=1  PParamMin=[]  PParamMax=[]  IParamMin=[]  IParamMax=[]  DParamMin=[]  DParamMax=[]  NParamMin=[]  NParamMax=[]  KbParamMin=[]  KbParamMax=[]  KtParamMin=[]  KtParamMax=[]  POutMin=[]  POutMax=[]  IOutMin=[]  IOutMax=[]  DOutMin=[]  DOutMax=[]  NOutMin=[]  NOutMax=[]  KbOutMin=[]  KbOutMax=[]  KtOutMin=[]  KtOutMax=[]  IntegratorOutMin=[]  IntegratorOutMax=[]  FilterOutMin=[]  FilterOutMax=[]  SumOutMin=[]  SumOutMax=[]  SumI1OutMin=[]  SumI1OutMax=[]  SumI2OutMin=[]  SumI2OutMax=[]  SumI3OutMin=[]  SumI3OutMax=[]  SumDOutMin=[]  SumDOutMax=[]  SaturationOutMin=[]  SaturationOutMax=[]  IntegratorContinuousStateAttributes=''  IntegratorStateMustResolveToSignalObject=off  IntegratorRTWStateStorageClass=Auto  FilterContinuousStateAttributes=''  FilterStateMustResolveToSignalObject=off  FilterRTWStateStorageClass=Auto  DifferentiatorICPrevScaledInput=0  DifferentiatorOutMin=[]  DifferentiatorOutMax=[]  FilterDiffOutCoefMin=[]  FilterDiffOutCoefMax=[]  SumDenOutMin=[]  SumDenOutMax=[]  SumNumOutMin=[]  SumNumOutMax=[]  ReciprocalOutMin=[]  ReciprocalOutMax=[]  DivideOutMin=[]  DivideOutMax=[]  TunerSelectOption=Transfer Function Based (PID Tuner App)
  cfblk{3,9,11,15} (4 alike) : Delay  DelayLengthSource=Input port
      settings: InputPortMap=u0,p1
  cfblk14 : simulink/Discrete/Tapped Delay  vinit=0.0  samptime=-1  NumDelays=1  DelayOrder=Oldest  includeCurrent=off
  cfblk16 : If  SampleTime=1
  cfblk18 : Subsystem  TreatAsAtomicUnit=on
  cfblk19 : Subsystem  TreatAsAtomicUnit=on
  cfblk{8,20..24} (6 alike) : Delay
  cfblk25 : DataTypeConversion  OutDataTypeStr=double
  cfblk26 : DataTypeConversion  OutDataTypeStr=double
  cfblk27 : DataTypeConversion  OutDataTypeStr=uint32
  cfblk28 : DataTypeConversion  OutDataTypeStr=double
  cfblk4 : DiscreteZeroPole  Poles=[0 0.5]  Gain=1  SampleTime=-1
  cfblk5 : DiscreteIntegrator  SampleTime=-1  OutDataTypeStr=double  ICPrevOutput=DiscIntNeverNeededParam  ICPrevScaledInput=DiscIntNeverNeededParam
  cfblk6 : DiscreteFir
  cyemi_{733,736..739,741,753..754,767,769,771,773,777..781} (17 alike) : DataTypeConversion  OutDataTypeStr=double
  cyemi_{734..735,740,742,766,768,770,772,774..776,782..783} (13 alike) : DataTypeConversion  OutDataTypeStr=uint32
  emi_{14,28,66,110,132,178,214,256} (8 alike) : UnaryMinus
  emi_111 : MATLAB Function  TreatAsAtomicUnit=on
  emi_133 : MATLAB Function  TreatAsAtomicUnit=on
  emi_15 : MATLAB Function  TreatAsAtomicUnit=on
  emi_179 : MATLAB Function  TreatAsAtomicUnit=on
  emi_215 : MATLAB Function  TreatAsAtomicUnit=on
  emi_257 : MATLAB Function  TreatAsAtomicUnit=on
  emi_29 : MATLAB Function  TreatAsAtomicUnit=on
  emi_67 : MATLAB Function  TreatAsAtomicUnit=on
  cfblk2 : Outport
  cfblk17 : Outport  Port=2
  wires:
  cfblk4/1 -> cyemi_753/1, cyemi_779/1
  cfblk11/1 -> cyemi_770/1, cyemi_772/1
  cfblk6/1 -> cfblk2/1
  cfblk19/1(cfblk2) -> cfblk17/1
  cfblk18/3(cfblk10) -> cyemi_735/1, cyemi_768/1
  cfblk16/1 -> cfblk18/Action
  cfblk16/2 -> cfblk19/Action
  cfblk27/1 -> cyemi_740/1, cyemi_742/1, cyemi_734/1
  cyemi_733/1 -> cfblk10/1
  cfblk5/1 -> cyemi_733/1
  cyemi_734/1 -> cfblk11/1
  cyemi_735/1 -> cfblk11/2
  cyemi_736/1 -> emi_132/1, emi_133/1(o), cfblk12/1
  cfblk25/1 -> cyemi_736/1
  cyemi_737/1 -> emi_178/1, emi_179/1(o), emi_214/1, emi_215/1(o), cfblk13/1
  cfblk28/1 -> cyemi_737/1
  cyemi_738/1 -> emi_110/1, emi_111/1(o), emi_67/1(o), cfblk14/1, emi_66/1
  cfblk18/2(cfblk9) -> cyemi_738/1
  cyemi_739/1 -> cfblk15/1
  cfblk8/1 -> cyemi_739/1
  cyemi_740/1 -> cfblk15/2
  cyemi_741/1 -> cfblk16/1
  cfblk21/1 -> cyemi_741/1
  cyemi_742/1 -> cfblk18/1(cfblk1)
  cyemi_753/1 -> cfblk19/1(cfblk1)
  cyemi_754/1 -> cfblk19/2(cfblk11)
  cfblk23/1 -> cyemi_754/1
  cyemi_766/1 -> cfblk20/1
  cfblk18/1(cfblk2) -> cyemi_766/1
  cyemi_767/1 -> emi_14/1, emi_15/1(o), cfblk21/1
  cfblk14/1 -> cyemi_767/1
  cyemi_768/1 -> cfblk22/1
  cyemi_769/1 -> cfblk23/1
  cfblk12/1 -> cyemi_769/1
  cyemi_770/1 -> cfblk24/1
  cyemi_771/1 -> cfblk25/1
  cfblk7/1 -> cyemi_771/1
  cyemi_772/1 -> cfblk26/1
  cyemi_773/1 -> cfblk27/1
  cfblk13/1 -> cyemi_773/1
  cyemi_774/1 -> cfblk28/1
  cfblk9/1 -> cyemi_774/1
  cyemi_775/1 -> cfblk3/1
  cfblk22/1 -> cyemi_775/1
  cyemi_776/1 -> cfblk3/2
  cfblk24/1 -> cyemi_776/1
  cyemi_777/1 -> cfblk4/1
  cfblk15/1 -> cyemi_777/1
  cyemi_778/1 -> cfblk5/1
  cfblk1/1 -> cyemi_778/1
  cyemi_779/1 -> cfblk6/1
  cyemi_780/1 -> emi_28/1, emi_29/1(o), cfblk7/1
  cfblk26/1 -> cyemi_780/1
  cyemi_781/1 -> emi_256/1, emi_257/1(o), cfblk8/1
  cfblk10/1 -> cyemi_781/1
  cyemi_782/1 -> cfblk9/1
  cfblk3/1 -> cyemi_782/1
  cyemi_783/1 -> cfblk9/2
  cfblk20/1 -> cyemi_783/1
  emi_14/1 -> emi_15/2(e)
  emi_28/1 -> emi_29/2(e)
  emi_66/1 -> emi_67/2(e)
  emi_110/1 -> emi_111/2(e)
  emi_132/1 -> emi_133/2(e)
  emi_178/1 -> emi_179/2(e)
  emi_214/1 -> emi_215/2(e)
  emi_256/1 -> emi_257/2(e)

== system sampleModel7424_pp_1_1/cfblk124/cfblk14 ==
  cfblk1 : Inport
  Action Port : ActionPort  ActionType=then
  cfblk3 : DiscreteFilter
  cfblk4 : DiscreteZeroPole  Poles=[0 0.5]  Gain=1  SampleTime=-1
  cfblk5 : UnitDelay  SampleTime=-1
  cfblk6 : DiscreteZeroPole  Poles=[0 0.5]  Gain=1  SampleTime=-1
  cyemi_{33..36} (4 alike) : DataTypeConversion  OutDataTypeStr=double
  cfblk2 : Outport
  cfblk7 : Outport  Port=2
  wires:
  cfblk1/1 -> cyemi_33/1, cyemi_36/1
  cfblk6/1 -> cfblk7/1
  cfblk4/1 -> cfblk2/1
  cyemi_33/1 -> cfblk3/1
  cyemi_34/1 -> cfblk4/1
  cfblk5/1 -> cyemi_34/1
  cyemi_35/1 -> cfblk5/1
  cfblk3/1 -> cyemi_35/1
  cyemi_36/1 -> cfblk6/1

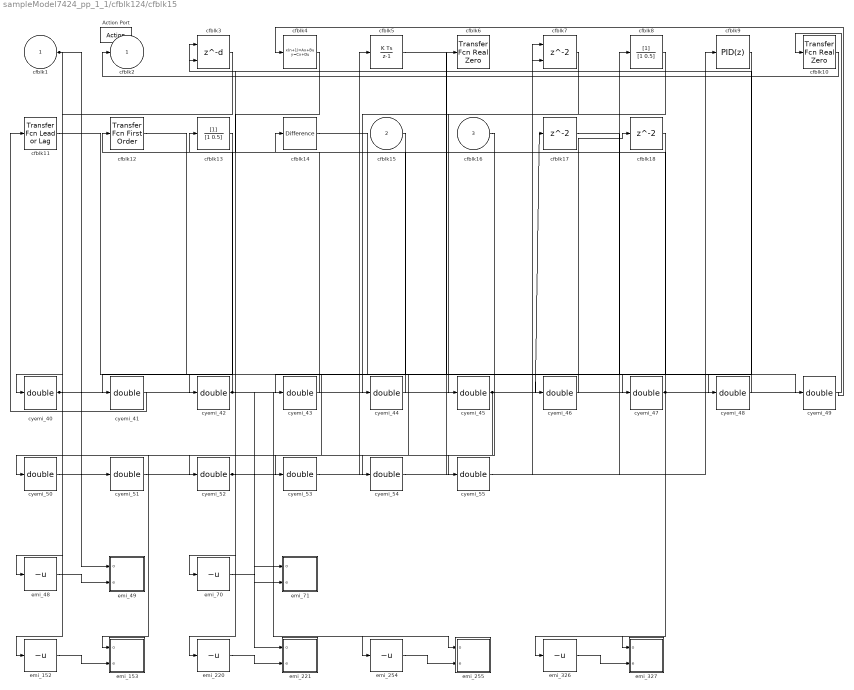
== system sampleModel7424_pp_1_1/cfblk124/cfblk15 ==
  cfblk1 : Inport
  cfblk15 : Inport  Port=2
  cfblk16 : Inport  Port=3
  Action Port : ActionPort  ActionType=else
  cfblk10 : simulink/Discrete/Transfer Fcn Real Zero  ZeroZ=0.75  ICPrevInput=0.0  DoSatur=off
      settings: SourceProductName=Simulink  SourceProductBaseCode=SL
  cfblk11 : simulink/Discrete/Transfer Fcn Lead or Lag  PoleZ=0.95  ZeroZ=0.75  ICPrevOutput=0.0  ICPrevInput=0.0  DoSatur=off
      settings: SourceProductName=Simulink  SourceProductBaseCode=SL
  cfblk12 : simulink/Discrete/Transfer Fcn First Order  PoleZ=0.95  ICPrevOutput=0.0  DoSatur=off
      settings: SourceProductName=Simulink
  cfblk13 : DiscreteFilter
  cfblk14 : simulink/Discrete/Difference  ICPrevInput=0.0  OutMin=[]  OutMax=[]  OutDataTypeStr=double  OutputDataTypeScalingMode=double  OutDataType=fixdt(1, 16)  OutScaling=2^-10  DoSatur=off
  cfblk17 : Delay
  cfblk18 : Delay
  cfblk3 : Delay  DelayLengthSource=Input port
      settings: InputPortMap=u0,p1
  cfblk4 : DiscreteStateSpace  SampleTime=-1
  cfblk5 : DiscreteIntegrator  SampleTime=-1  OutDataTypeStr=double  ICPrevOutput=DiscIntNeverNeededParam  ICPrevScaledInput=DiscIntNeverNeededParam
  cfblk6 : simulink/Discrete/Transfer Fcn Real Zero  ZeroZ=0.75  ICPrevInput=0.0  DoSatur=off
      settings: SourceProductName=Simulink  SourceProductBaseCode=SL
  cfblk7 : Delay  ShowEnablePort=on
      settings: InputPortMap=u0,e6
  cfblk8 : DiscreteFilter
  cfblk9 : simulink/Continuous/PID Controller  Controller=PID  TimeDomain=Discrete-time  SampleTime=-1  IntegratorMethod=Forward Euler  FilterMethod=Forward Euler  Form=Parallel  UseFilter=on  ControllerParametersSource=internal  P=1  I=1  D=0  N=100  InitialConditionSource=internal  InitialConditionForIntegrator=0  InitialConditionForFilter=0  ExternalReset=none  LimitOutput=off  UpperSaturationLimit=inf  LowerSaturationLimit=-inf  LinearizeAsGain=off  AntiWindupMode=none  Kb=1  TrackingMode=off  Kt=1  PParamMin=[]  PParamMax=[]  IParamMin=[]  IParamMax=[]  DParamMin=[]  DParamMax=[]  NParamMin=[]  NParamMax=[]  KbParamMin=[]  KbParamMax=[]  KtParamMin=[]  KtParamMax=[]  POutMin=[]  POutMax=[]  IOutMin=[]  IOutMax=[]  DOutMin=[]  DOutMax=[]  NOutMin=[]  NOutMax=[]  KbOutMin=[]  KbOutMax=[]  KtOutMin=[]  KtOutMax=[]  IntegratorOutMin=[]  IntegratorOutMax=[]  FilterOutMin=[]  FilterOutMax=[]  SumOutMin=[]  SumOutMax=[]  SumI1OutMin=[]  SumI1OutMax=[]  SumI2OutMin=[]  SumI2OutMax=[]  SumI3OutMin=[]  SumI3OutMax=[]  SumDOutMin=[]  SumDOutMax=[]  SaturationOutMin=[]  SaturationOutMax=[]  IntegratorContinuousStateAttributes=''  IntegratorStateMustResolveToSignalObject=off  IntegratorRTWStateStorageClass=Auto  FilterContinuousStateAttributes=''  FilterStateMustResolveToSignalObject=off  FilterRTWStateStorageClass=Auto  DifferentiatorICPrevScaledInput=0  DifferentiatorOutMin=[]  DifferentiatorOutMax=[]  FilterDiffOutCoefMin=[]  FilterDiffOutCoefMax=[]  SumDenOutMin=[]  SumDenOutMax=[]  SumNumOutMin=[]  SumNumOutMax=[]  ReciprocalOutMin=[]  ReciprocalOutMax=[]  DivideOutMin=[]  DivideOutMax=[]  TunerSelectOption=Transfer Function Based (PID Tuner App)
  cyemi_{40..55} (16 alike) : DataTypeConversion  OutDataTypeStr=double
  emi_{48,70,152,220,254,326} (6 alike) : UnaryMinus
  emi_153 : MATLAB Function  TreatAsAtomicUnit=on
  emi_221 : MATLAB Function  TreatAsAtomicUnit=on
  emi_255 : MATLAB Function  TreatAsAtomicUnit=on
  emi_327 : MATLAB Function  TreatAsAtomicUnit=on
  emi_49 : MATLAB Function  TreatAsAtomicUnit=on
  emi_71 : MATLAB Function  TreatAsAtomicUnit=on
  cfblk2 : Outport
  wires:
  cfblk1/1 -> cyemi_50/1, cyemi_51/1
  cfblk10/1 -> cfblk2/1
  cyemi_40/1 -> cfblk10/1, emi_48/1, emi_49/1(o)
  cfblk3/1 -> cyemi_40/1
  cyemi_41/1 -> cfblk11/1
  cfblk13/1 -> cyemi_41/1
  cyemi_42/1 -> cfblk12/1, emi_70/1, emi_71/1(o), emi_254/1, emi_255/1(o)
  cfblk11/1 -> cyemi_42/1
  cyemi_43/1 -> cfblk13/1
  cfblk15/1 -> cyemi_43/1
  cyemi_44/1 -> cfblk14/1
  cfblk8/1 -> cyemi_44/1
  cyemi_45/1 -> cfblk17/1, emi_152/1, emi_153/1(o)
  cfblk7/1 -> cyemi_45/1
  cyemi_46/1 -> cfblk18/1
  cfblk14/1 -> cyemi_46/1
  cyemi_47/1 -> cfblk3/1, emi_326/1, emi_327/1(o)
  cfblk5/1 -> cyemi_47/1
  cyemi_48/1 -> cfblk3/2
  cfblk12/1 -> cyemi_48/1
  cyemi_49/1 -> cfblk4/1
  cfblk17/1 -> cyemi_49/1
  cyemi_50/1 -> cfblk5/1
  cyemi_51/1 -> cfblk6/1
  cyemi_52/1 -> cfblk7/1, emi_220/1, emi_221/1(o)
  cfblk4/1 -> cyemi_52/1
  cyemi_53/1 -> cfblk7/2
  cfblk9/1 -> cyemi_53/1
  cyemi_54/1 -> cfblk8/1
  cfblk18/1 -> cyemi_54/1
  cyemi_55/1 -> cfblk9/1
  cfblk16/1 -> cyemi_55/1
  emi_48/1 -> emi_49/2(e)
  emi_70/1 -> emi_71/2(e)
  emi_152/1 -> emi_153/2(e)
  emi_220/1 -> emi_221/2(e)
  emi_254/1 -> emi_255/2(e)
  emi_326/1 -> emi_327/2(e)

== system sampleModel7424_pp_1_1/cfblk124/cfblk16 ==
  cfblk1 : Inport
  cfblk11 : Inport  Port=2
  cfblk12 : Inport  Port=3
  cfblk13 : Inport  Port=4
  cfblk14 : Inport  Port=5
  Action Port : ActionPort  ActionType=then
  cfblk10 : simulink/Discrete/Transfer Fcn First Order  PoleZ=0.95  ICPrevOutput=0.0  DoSatur=off
      settings: SourceProductName=Simulink
  cfblk15 : Delay
  cfblk16 : Delay
  cfblk3 : DiscreteFir
  cfblk4 : Delay  DelayLengthSource=Input port
      settings: InputPortMap=u0,p1
  cfblk5 : DiscreteStateSpace  SampleTime=-1
  cfblk6 : simulink/Discrete/Transfer Fcn Real Zero  ZeroZ=0.75  ICPrevInput=0.0  DoSatur=off
      settings: SourceProductName=Simulink  SourceProductBaseCode=SL
  cfblk7 : Delay  ShowEnablePort=on
      settings: InputPortMap=u0,e6
  cfblk8 : simulink/Discrete/Transfer Fcn Real Zero  ZeroZ=0.75  ICPrevInput=0.0  DoSatur=off
      settings: SourceProductName=Simulink  SourceProductBaseCode=SL
  cfblk9 : Delay
  cyemi_{61..72} (12 alike) : DataTypeConversion  OutDataTypeStr=double
  cfblk2 : Outport
  wires:
  cfblk1/1 -> cfblk2/1
  cyemi_61/1 -> cfblk10/1
  cfblk13/1 -> cyemi_61/1
  cyemi_62/1 -> cfblk15/1
  cfblk7/1 -> cyemi_62/1
  cyemi_63/1 -> cfblk16/1
  cfblk6/1 -> cyemi_63/1
  cyemi_64/1 -> cfblk3/1
  cfblk12/1 -> cyemi_64/1
  cyemi_65/1 -> cfblk4/1
  cfblk14/1 -> cyemi_65/1
  cyemi_66/1 -> cfblk4/2
  cfblk15/1 -> cyemi_66/1
  cyemi_67/1 -> cfblk5/1
  cfblk16/1 -> cyemi_67/1
  cyemi_68/1 -> cfblk6/1
  cfblk5/1 -> cyemi_68/1
  cyemi_69/1 -> cfblk7/1
  cfblk11/1 -> cyemi_69/1
  cyemi_70/1 -> cfblk7/2
  cfblk9/1 -> cyemi_70/1
  cyemi_71/1 -> cfblk8/1
  cfblk10/1 -> cyemi_71/1
  cyemi_72/1 -> cfblk9/1
  cfblk4/1 -> cyemi_72/1

== system sampleModel7424_pp_1_1/cfblk124/cfblk17 ==
  cfblk1 : Inport
  cfblk12 : Inport  Port=2
  cfblk13 : Inport  Port=3
  cfblk14 : Inport  Port=4
  cfblk15 : Inport  Port=5
  Action Port : ActionPort  ActionType=else
  cfblk10 : DiscreteFilter
  cfblk11 : simulink/Discrete/Transfer Fcn Real Zero  ZeroZ=0.75  ICPrevInput=0.0  DoSatur=off
      settings: SourceProductName=Simulink  SourceProductBaseCode=SL
  cfblk16 : Delay
  cfblk3 : DiscreteFilter
  cfblk4 : DiscreteZeroPole  Poles=[0 0.5]  Gain=1  SampleTime=-1
  cfblk5 : simulink/Discrete/Transfer Fcn Real Zero  ZeroZ=0.75  ICPrevInput=0.0  DoSatur=off
      settings: SourceProductName=Simulink  SourceProductBaseCode=SL
  cfblk6 : UnitDelay  SampleTime=-1
  cfblk7 : simulink/Discrete/Transfer Fcn Real Zero  ZeroZ=0.75  ICPrevInput=0.0  DoSatur=off
      settings: SourceProductName=Simulink  SourceProductBaseCode=SL
  cfblk8 : DiscreteFir
  cfblk9 : simulink/Continuous/PID Controller  Controller=PID  TimeDomain=Discrete-time  SampleTime=-1  IntegratorMethod=Forward Euler  FilterMethod=Forward Euler  Form=Parallel  UseFilter=on  ControllerParametersSource=internal  P=1  I=1  D=0  N=100  InitialConditionSource=internal  InitialConditionForIntegrator=0  InitialConditionForFilter=0  ExternalReset=none  LimitOutput=off  UpperSaturationLimit=inf  LowerSaturationLimit=-inf  LinearizeAsGain=off  AntiWindupMode=none  Kb=1  TrackingMode=off  Kt=1  PParamMin=[]  PParamMax=[]  IParamMin=[]  IParamMax=[]  DParamMin=[]  DParamMax=[]  NParamMin=[]  NParamMax=[]  KbParamMin=[]  KbParamMax=[]  KtParamMin=[]  KtParamMax=[]  POutMin=[]  POutMax=[]  IOutMin=[]  IOutMax=[]  DOutMin=[]  DOutMax=[]  NOutMin=[]  NOutMax=[]  KbOutMin=[]  KbOutMax=[]  KtOutMin=[]  KtOutMax=[]  IntegratorOutMin=[]  IntegratorOutMax=[]  FilterOutMin=[]  FilterOutMax=[]  SumOutMin=[]  SumOutMax=[]  SumI1OutMin=[]  SumI1OutMax=[]  SumI2OutMin=[]  SumI2OutMax=[]  SumI3OutMin=[]  SumI3OutMax=[]  SumDOutMin=[]  SumDOutMax=[]  SaturationOutMin=[]  SaturationOutMax=[]  IntegratorContinuousStateAttributes=''  IntegratorStateMustResolveToSignalObject=off  IntegratorRTWStateStorageClass=Auto  FilterContinuousStateAttributes=''  FilterStateMustResolveToSignalObject=off  FilterRTWStateStorageClass=Auto  DifferentiatorICPrevScaledInput=0  DifferentiatorOutMin=[]  DifferentiatorOutMax=[]  FilterDiffOutCoefMin=[]  FilterDiffOutCoefMax=[]  SumDenOutMin=[]  SumDenOutMax=[]  SumNumOutMin=[]  SumNumOutMax=[]  ReciprocalOutMin=[]  ReciprocalOutMax=[]  DivideOutMin=[]  DivideOutMax=[]  TunerSelectOption=Transfer Function Based (PID Tuner App)
  cyemi_{78..87} (10 alike) : DataTypeConversion  OutDataTypeStr=double
  emi_112 : UnaryMinus
  emi_113 : MATLAB Function  TreatAsAtomicUnit=on
  emi_300 : UnaryMinus
  emi_301 : MATLAB Function  TreatAsAtomicUnit=on
  emi_322 : UnaryMinus
  emi_323 : MATLAB Function  TreatAsAtomicUnit=on
  cfblk2 : Outport
  wires:
  cfblk3/1 -> cfblk2/1
  cyemi_78/1 -> cfblk10/1
  cfblk14/1 -> cyemi_78/1
  cyemi_79/1 -> cfblk11/1, emi_322/1, emi_323/1(o)
  cfblk4/1 -> cyemi_79/1
  cyemi_80/1 -> cfblk16/1
  cfblk7/1 -> cyemi_80/1
  cyemi_81/1 -> cfblk3/1
  cfblk5/1 -> cyemi_81/1
  cyemi_82/1 -> cfblk4/1
  cfblk16/1 -> cyemi_82/1
  cyemi_83/1 -> cfblk5/1, emi_112/1, emi_113/1(o)
  cfblk13/1 -> cyemi_83/1
  cyemi_84/1 -> cfblk6/1
  cfblk9/1 -> cyemi_84/1
  cyemi_85/1 -> cfblk7/1, emi_300/1, emi_301/1(o)
  cfblk6/1 -> cyemi_85/1
  cyemi_86/1 -> cfblk8/1
  cfblk15/1 -> cyemi_86/1
  cyemi_87/1 -> cfblk9/1
  cfblk11/1 -> cyemi_87/1
  emi_112/1 -> emi_113/2(e)
  emi_300/1 -> emi_301/2(e)
  emi_322/1 -> emi_323/2(e)

== system sampleModel7424_pp_1_1/cfblk125/cfblk11 ==
  cfblk1 : Inport
  cfblk12 : Inport  Port=2
  Action Port : ActionPort  ActionType=then
  cfblk10 : DiscreteFilter
  cfblk11 : simulink/Discrete/Transfer Fcn Real Zero  ZeroZ=0.75  ICPrevInput=0.0  DoSatur=off
      settings: SourceProductName=Simulink  SourceProductBaseCode=SL
  cfblk15 : Delay
  cfblk16 : DataTypeConversion  OutDataTypeStr=uint32
  cfblk17 : DataTypeConversion  OutDataTypeStr=double
  cfblk3 : DiscreteFir
  cfblk4 : simulink/Continuous/PID Controller  Controller=PID  TimeDomain=Discrete-time  SampleTime=-1  IntegratorMethod=Forward Euler  FilterMethod=Forward Euler  Form=Parallel  UseFilter=on  ControllerParametersSource=internal  P=1  I=1  D=0  N=100  InitialConditionSource=internal  InitialConditionForIntegrator=0  InitialConditionForFilter=0  ExternalReset=none  LimitOutput=off  UpperSaturationLimit=inf  LowerSaturationLimit=-inf  LinearizeAsGain=off  AntiWindupMode=none  Kb=1  TrackingMode=off  Kt=1  PParamMin=[]  PParamMax=[]  IParamMin=[]  IParamMax=[]  DParamMin=[]  DParamMax=[]  NParamMin=[]  NParamMax=[]  KbParamMin=[]  KbParamMax=[]  KtParamMin=[]  KtParamMax=[]  POutMin=[]  POutMax=[]  IOutMin=[]  IOutMax=[]  DOutMin=[]  DOutMax=[]  NOutMin=[]  NOutMax=[]  KbOutMin=[]  KbOutMax=[]  KtOutMin=[]  KtOutMax=[]  IntegratorOutMin=[]  IntegratorOutMax=[]  FilterOutMin=[]  FilterOutMax=[]  SumOutMin=[]  SumOutMax=[]  SumI1OutMin=[]  SumI1OutMax=[]  SumI2OutMin=[]  SumI2OutMax=[]  SumI3OutMin=[]  SumI3OutMax=[]  SumDOutMin=[]  SumDOutMax=[]  SaturationOutMin=[]  SaturationOutMax=[]  IntegratorContinuousStateAttributes=''  IntegratorStateMustResolveToSignalObject=off  IntegratorRTWStateStorageClass=Auto  FilterContinuousStateAttributes=''  FilterStateMustResolveToSignalObject=off  FilterRTWStateStorageClass=Auto  DifferentiatorICPrevScaledInput=0  DifferentiatorOutMin=[]  DifferentiatorOutMax=[]  FilterDiffOutCoefMin=[]  FilterDiffOutCoefMax=[]  SumDenOutMin=[]  SumDenOutMax=[]  SumNumOutMin=[]  SumNumOutMax=[]  ReciprocalOutMin=[]  ReciprocalOutMax=[]  DivideOutMin=[]  DivideOutMax=[]  TunerSelectOption=Transfer Function Based (PID Tuner App)
  cfblk5 : DiscreteFir
  cfblk6 : Delay  DelayLengthSource=Input port
      settings: InputPortMap=u0,p1
  cfblk7 : DiscreteZeroPole  Poles=[0 0.5]  Gain=1  SampleTime=-1
  cfblk8 : simulink/Discrete/Tapped Delay  vinit=0.0  samptime=-1  NumDelays=1  DelayOrder=Oldest  includeCurrent=off
  cfblk9 : DiscreteFilter
  cyemi_{114..122,124..126} (12 alike) : DataTypeConversion  OutDataTypeStr=double
  cyemi_123 : DataTypeConversion  OutDataTypeStr=uint32
  cfblk2 : Outport
  cfblk13 : Outport  Port=2
  cfblk14 : Outport  Port=3
  wires:
  cfblk5/1 -> cfblk14/1
  cfblk4/1 -> cfblk13/1
  cfblk7/1 -> cfblk2/1, cyemi_115/1
  cfblk3/1 -> cyemi_118/1, cyemi_125/1
  cyemi_114/1 -> cfblk10/1
  cfblk17/1 -> cyemi_114/1
  cyemi_115/1 -> cfblk11/1
  cyemi_116/1 -> cfblk15/1
  cfblk9/1 -> cyemi_116/1
  cyemi_117/1 -> cfblk16/1
  cfblk10/1 -> cyemi_117/1
  cyemi_118/1 -> cfblk17/1
  cyemi_119/1 -> cfblk3/1
  cfblk15/1 -> cyemi_119/1
  cyemi_120/1 -> cfblk4/1
  cfblk1/1 -> cyemi_120/1
  cyemi_121/1 -> cfblk5/1
  cfblk6/1 -> cyemi_121/1
  cyemi_122/1 -> cfblk6/1
  cfblk11/1 -> cyemi_122/1
  cyemi_123/1 -> cfblk6/2
  cfblk16/1 -> cyemi_123/1
  cyemi_124/1 -> cfblk7/1
  cfblk12/1 -> cyemi_124/1
  cyemi_125/1 -> cfblk8/1
  cyemi_126/1 -> cfblk9/1
  cfblk8/1 -> cyemi_126/1
